simulink model "watertank"  (R2023a)
settings: Solver=VariableStepAuto  StartTime=0.0  StopTime=10.0  RelTol=1e-3
settings Model: Creator=yaboi  LastModifiedBy=yaboi

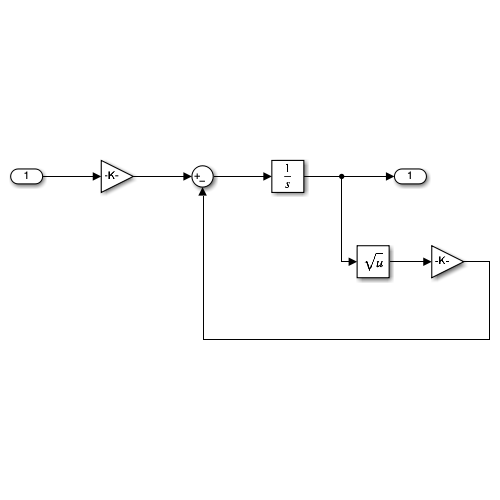
[thumbnail: Simulink's stored preview of the top-level diagram]
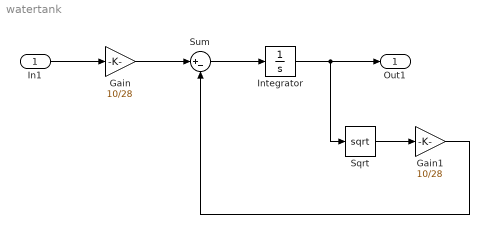
== system watertank ==
  In1 : Inport
  Gain : Gain  Gain=10/28
  Gain1 : Gain  Gain=10/28
  Integrator : Integrator  InitialCondition=2
  Sqrt : Sqrt
  Sum : Sum  Inputs=|+-
  Out1 : Outport
  wires:
  In1/1 -> Gain/1
  Gain/1 -> Sum/1
  Sum/1 -> Integrator/1
  Integrator/1 -> Sqrt/1, Out1/1
  Sqrt/1 -> Gain1/1
  Gain1/1 -> Sum/2
